simulink model "gm_HDLPayloadFull_vs"  (R2024a)
settings: Solver=FixedStepDiscrete  StartTime=0.0  StopTime=stopTime  RelTol=1e-3
values from neighbouring files (symbols this model uses):
  blockSize = logical([0 0])    [testPayloadFull.m]
  dataChars = uint8(zeros(payloadLenInWords, 1))    [testPayloadFull.m]
  fecRate = logical([1 0 0])    [testPayloadFull.m]
  fs = 1    [testPayloadFull.m]
  scramblerInit = logical([1 1 0 0])    [testPayloadFull.m]
undefined symbols (not defined in the file or in its folder): batId, clk, clk_enable, numDataCarriers, payloadWordsPerBlock0, psduSize, repNumber, reset_x
libraries: hdlmdlgenlib x65, hdlsllib x39, simulink x7, whdlutilities x4, dspsrcs4 x2, whdledac x1, vivadosimlib x1
settings Model: Creator=cotti  LastModifiedBy=cotti
settings OptimizationCC: BlockReduction=off  ConditionallyExecuteInputs=off  DefaultParameterBehavior=Inlined  InheritOutputTypeSmallerThanSingle=on
settings DebuggingCC: AlgebraicLoopMsg=error  ArtificialAlgebraicLoopMsg=error  InheritedTsInSrcMsg=none  SingleTaskRateTransMsg=error  UnconnectedInputMsg=warning  UnconnectedOutputMsg=warning  UnconnectedLineMsg=warning
settings HardwareCC: ProdBitPerPointer=32  ProdBitPerSizeT=32  ProdBitPerPtrDiffT=32  ProdLargestAtomicFloat=None  ProdIntDivRoundTo=Undefined  ProdEndianess=Unspecified  ProdWordSize=32  ProdHWDeviceType=ASIC/FPGA->ASIC/FPGA  TargetBitPerLong=64  TargetBitPerPointer=64  TargetBitPerSizeT=64  TargetBitPerPtrDiffT=64  TargetLongLongMode=on  TargetIntDivRoundTo=Zero  TargetEndianess=LittleEndian  TargetWordSize=64  TargetHWDeviceType=Custom Processor->MATLAB Host Computer  ProdEqTarget=off

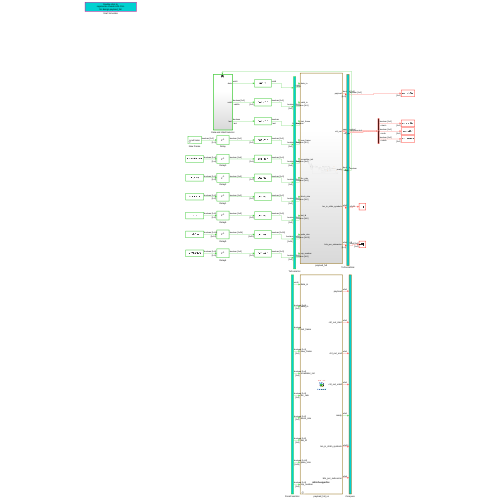
[thumbnail: Simulink's stored preview of the top-level diagram]
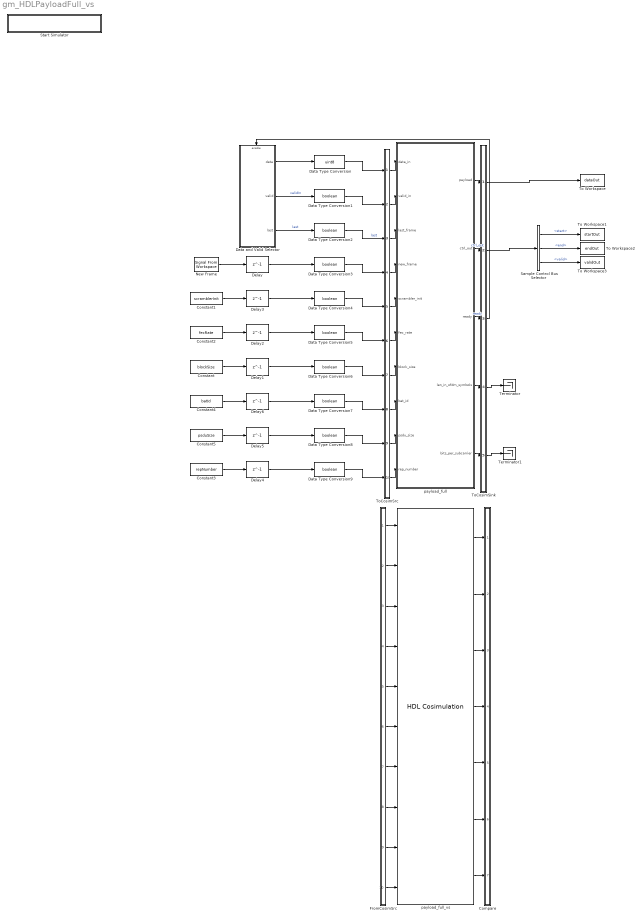
== system gm_HDLPayloadFull_vs ==
  Compare : Subsystem
      mask Display: disp('')
  Constant : Constant  Value=blockSize  VectorParams1D=off  OutDataTypeStr=boolean  SampleTime=1/fs
  Constant1 : Constant  Value=scramblerInit  VectorParams1D=off  OutDataTypeStr=boolean  SampleTime=1/fs
  Constant2 : Constant  Value=fecRate  VectorParams1D=off  OutDataTypeStr=boolean  SampleTime=1/fs
  Constant3 : Constant  Value=repNumber  VectorParams1D=off  OutDataTypeStr=boolean  SampleTime=1/fs
  Constant4 : Constant  Value=batId  VectorParams1D=off  OutDataTypeStr=boolean  SampleTime=1/fs
  Constant5 : Constant  Value=psduSize  VectorParams1D=off  OutDataTypeStr=boolean  SampleTime=1/fs
  Data Type Conversion : DataTypeConversion  OutDataTypeStr=uint8  SaturateOnIntegerOverflow=off  RndMeth=Floor
  Data Type Conversion{1..9} (9 alike) : DataTypeConversion  OutDataTypeStr=boolean  SaturateOnIntegerOverflow=off  RndMeth=Floor
  Data and Valid Selector : Subsystem  TreatAsAtomicUnit=on
  Delay{,1..6} (7 alike) : Delay  DelayLength=1  InitialCondition=0  UseCircularBuffer=on
  FromCosimSrc : Subsystem
      mask Display: disp('')
  New Frame : dspsrcs4/Signal From Workspace  X=newFrame  Ts=1/fs  nsamps=1  OutputAfterFinalValue=Setting to zero  ignoreOrWarnInputAndFrameLengths=off  OutputFrames=off
  Sample Control Bus Selector : whdlutilities/Sample Control Bus Selector  OutputSignals=start,end,valid
  Start Simulator : Subsystem
      settings: OpenFcn=|
      | cosimDirName = pwd;
      | cd 'hdl_prj/hdlsrc/HDLPayloadFull';
      | [s,r] = system('vivado -mode batch -source gm_HDLPayloadFull_vs.tcl','-echo');
      | cd (cosimDirName);
      | clear cosimDirName;
      | if s
      |    error('Failed to create Vivado HDL design DLL using script gm_HDLPayloadFull_vs.tcl.');
      | end
      mask Display: disp('Double-click to\nregenerate Vivado HDL DLL\nfor design payload_full')
  Terminator : Terminator
  Terminator1 : Terminator
  To Workspace : ToWorkspace  VariableName=dataOut  SampleTime=1/(8*fs)
      settings: Save2DSignal=2-D array (concatenate along first dimension)
  To Workspace1 : ToWorkspace  VariableName=startOut  SampleTime=1/(8*fs)
      settings: Save2DSignal=2-D array (concatenate along first dimension)
  To Workspace2 : ToWorkspace  VariableName=endOut  SampleTime=1/(8*fs)
      settings: Save2DSignal=2-D array (concatenate along first dimension)
  To Workspace3 : ToWorkspace  VariableName=validOut  SampleTime=1/(8*fs)
      settings: Save2DSignal=2-D array (concatenate along first dimension)
  ToCosimSink : Subsystem
      mask Display: disp('')
  ToCosimSrc : Subsystem
      mask Display: disp('')
  payload_full : Subsystem
  payload_full_vs : vivadosimlib/HDL Cosimulation  PortPaths=/payload_full/data_in;/payload_full/valid_in;/payload_full/last_frame;/payload_full/new_frame;/payload_full/scrambler_init;/payload_full/fec_rate;/payload_full/block_size;/payload_full/bat_id;/payload_full/psdu_size;/payload_full/rep_number;/payload_full/payload;/payload_full/ctrl_out_start;/payload_full/ctrl_out_end;/payload_full/ctrl_out_valid;/payload_full/ready;/payload_full/len_in_ofdm_symbols;/payload_full/bits_per_subcarrier  PortModes=[1 1 1 1 1 1 1 1 1 1 2 2 2 2 2 2 2 ]  PortTimes=[-1 -1 -1 -1 -1 -1 -1 -1 -1 -1 0.125 0.125 0.125 0.125 1 0.125 0.125 ]  PortSigns=[-1 -1 -1 -1 -1 -1 -1 -1 -1 -1 0 0 0 0 0 0 0 ]  PortFracLengths=[0,0,0,0,0,0,0,0,0,0,0,0,0,0,0,0,0]  PortWordLengths=[-1,-1,-1,-1,-1,-1,-1,-1,-1,-1,1,1,1,1,1,29,4]  PortHDLWordSizes=[8,1,1,1,1,1,1,1,1,1,1,1,1,1,1,29,4]  CommLocal=on  CommSharedMemory=on  CommPortNumber=4449  CommShowInfo=on  ClockPaths=clk;clk_enable;reset_x;  ClockModes=[2 4 3]  ClockTimes=[1e-08 3.7e-08 2.7e-08]  TclPostSimCommand="puts \"done\""  TimingMode=ns  TimingScaleFactor=80  idxCellArray={'UNUSED_VAR'}  CosimBypass=Full Simulation  AllowDirectFeedthrough=on  ProductName=EDA Simulator Link VS  RunAutoTimescale=off  HdlClocks=0  PreRunTime=40  PreRunTimeUnit=ns
  wires:
  Constant3/1 -> Delay4/1
  Delay1/1 -> Data Type Conversion6/1
  Sample Control Bus Selector/1 -> To Workspace1/1  "<start>"
  Constant5/1 -> Delay5/1
  New Frame/1 -> Delay/1
  Sample Control Bus Selector/3 -> To Workspace3/1  "<valid>"
  Sample Control Bus Selector/2 -> To Workspace2/1  "<end>"
  Delay5/1 -> Data Type Conversion8/1
  Constant4/1 -> Delay6/1
  Delay2/1 -> Data Type Conversion5/1
  Data and Valid Selector/3(last) -> Data Type Conversion2/1  "last"
  Constant2/1 -> Delay2/1
  Delay3/1 -> Data Type Conversion4/1
  Constant1/1 -> Delay3/1
  Delay/1 -> Data Type Conversion3/1
  Data and Valid Selector/1(data) -> Data Type Conversion/1
  Data and Valid Selector/2(valid) -> Data Type Conversion1/1  "validIn"
  Delay4/1 -> Data Type Conversion9/1
  Constant/1 -> Delay1/1
  Delay6/1 -> Data Type Conversion7/1
  ToCosimSrc/1(out1) -> payload_full/1(data_in)
  ToCosimSrc/2(out2) -> payload_full/2(valid_in)
  ToCosimSrc/3(out3) -> payload_full/3(last_frame)
  ToCosimSrc/4(out4) -> payload_full/4(new_frame)
  ToCosimSrc/5(out5) -> payload_full/5(scrambler_init)
  ToCosimSrc/6(out6) -> payload_full/6(fec_rate)
  ToCosimSrc/7(out7) -> payload_full/7(block_size)
  ToCosimSrc/8(out8) -> payload_full/8(bat_id)
  ToCosimSrc/9(out9) -> payload_full/9(psdu_size)
  ToCosimSrc/10(out10) -> payload_full/10(rep_number)
  payload_full/1(payload) -> ToCosimSink/1(in1)
  payload_full/2(ctrl_out) -> ToCosimSink/2(in2)  "ctrl_out"
  payload_full/3(ready) -> ToCosimSink/3(in3)  "ready"
  payload_full/4(len_in_ofdm_symbols) -> ToCosimSink/4(in4)
  payload_full/5(bits_per_subcarrier) -> ToCosimSink/5(in5)
  Data Type Conversion/1 -> ToCosimSrc/1(in1)
  Data Type Conversion1/1 -> ToCosimSrc/2(in2)
  Data Type Conversion2/1 -> ToCosimSrc/3(in3)  "last"
  Data Type Conversion3/1 -> ToCosimSrc/4(in4)
  Data Type Conversion4/1 -> ToCosimSrc/5(in5)
  Data Type Conversion5/1 -> ToCosimSrc/6(in6)
  Data Type Conversion6/1 -> ToCosimSrc/7(in7)
  Data Type Conversion7/1 -> ToCosimSrc/8(in8)
  Data Type Conversion8/1 -> ToCosimSrc/9(in9)
  Data Type Conversion9/1 -> ToCosimSrc/10(in10)
  ToCosimSink/1(out1) -> To Workspace/1
  ToCosimSink/2(out2) -> Sample Control Bus Selector/1
  ToCosimSink/3(out3) -> Data and Valid Selector/Enable
  ToCosimSink/4(out4) -> Terminator/1
  ToCosimSink/5(out5) -> Terminator1/1
  FromCosimSrc/1(out1) -> payload_full_vs/1
  FromCosimSrc/2(out2) -> payload_full_vs/2
  FromCosimSrc/3(out3) -> payload_full_vs/3
  FromCosimSrc/4(out4) -> payload_full_vs/4
  FromCosimSrc/5(out5) -> payload_full_vs/5
  FromCosimSrc/6(out6) -> payload_full_vs/6
  FromCosimSrc/7(out7) -> payload_full_vs/7
  FromCosimSrc/8(out8) -> payload_full_vs/8
  FromCosimSrc/9(out9) -> payload_full_vs/9
  FromCosimSrc/10(out10) -> payload_full_vs/10
  payload_full_vs/1 -> Compare/1(in1)
  payload_full_vs/2 -> Compare/2(in2)
  payload_full_vs/3 -> Compare/3(in3)
  payload_full_vs/4 -> Compare/4(in4)
  payload_full_vs/5 -> Compare/5(in5)
  payload_full_vs/6 -> Compare/6(in6)
  payload_full_vs/7 -> Compare/7(in7)

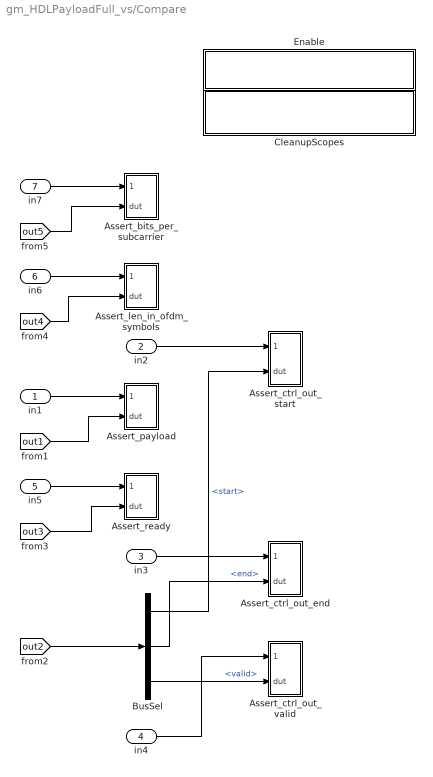
== system gm_HDLPayloadFull_vs/Compare ==
  in1 : Inport
  in2 : Inport  Port=2
  in3 : Inport  Port=3
  in4 : Inport  Port=4
  in5 : Inport  Port=5
  in6 : Inport  Port=6
  in7 : Inport  Port=7
  Assert_bits_per_subcarrier : Subsystem
      settings: LibrarySourceBlock=hdlmdlgenlib/AssertEq
  Assert_ctrl_out_end : Subsystem
      settings: LibrarySourceBlock=hdlmdlgenlib/AssertEq
  Assert_ctrl_out_start : Subsystem
      settings: LibrarySourceBlock=hdlmdlgenlib/AssertEq
  Assert_ctrl_out_valid : Subsystem
      settings: LibrarySourceBlock=hdlmdlgenlib/AssertEq
  Assert_len_in_ofdm_symbols : Subsystem
      settings: LibrarySourceBlock=hdlmdlgenlib/AssertEq
  Assert_payload : Subsystem
      settings: LibrarySourceBlock=hdlmdlgenlib/AssertEq
  Assert_ready : Subsystem
      settings: LibrarySourceBlock=hdlmdlgenlib/AssertEq
  BusSel : BusSelector  OutputSignals=start,end,valid
  CleanupScopes : Subsystem
      settings: OpenFcn=|
      | blkName = gcb; %self block
      | idx = regexp(blkName, '/CleanupScopes$', 'once');
      | blkParent = blkName(1:idx-1);
      | blks=find_system(blkParent, 'LookUnderMasks', 'all','blocktype', 'Scope');
      | for itr = 1:length(blks)
      | 	 hScopeCfg = get_param(blks{itr},'ScopeConfiguration');
      | 	 hScopeCfg.Visible = ~ hScopeCfg.Visible;
      | end
      | drawnow;
      mask Display: fprintf(message('hdlcoder:cosim:vnl_dblclick').getString());
  Enable : Subsystem
      settings: OpenFcn=|
      | blkName = gcb;
      | idx = regexp(blkName, '/Enable$', 'once');
      | blkParent = blkName(1:idx-1);
      | blks=find_system(blkParent, 'LookUnderMasks', 'all','blocktype', 'Assertion');
      | e = get_param(blks{1}, 'Enabled');
      | if strcmp(e, 'on'), f= 'off';, else, f = 'on';, end
      | for ii=1:length(blks), set_param(blks{ii}, 'Enabled', f);, end
      | set_param(gcb, 'MaskDisplay',['fprintf(message(''hdlcoder:cosim:vnl_dblclick_assertions'',','''',upper(e),'''',').getString())']);
      mask Display: fprintf(message('hdlcoder:cosim:vnl_dblclick_assertions','OFF').getString());
  wires:
  in4/1 -> Assert_ctrl_out_valid/1(cosim)
  in6/1 -> Assert_len_in_ofdm_symbols/1(cosim)
  in7/1 -> Assert_bits_per_subcarrier/1(cosim)
  [out5] -> Assert_bits_per_subcarrier/2(dut)
  [out4] -> Assert_len_in_ofdm_symbols/2(dut)
  in1/1 -> Assert_payload/1(cosim)
  in5/1 -> Assert_ready/1(cosim)
  [out1] -> Assert_payload/2(dut)
  [out3] -> Assert_ready/2(dut)
  [out2] -> BusSel/1
  BusSel/1 -> Assert_ctrl_out_start/2(dut)  "<start>"
  BusSel/3 -> Assert_ctrl_out_valid/2(dut)  "<valid>"
  BusSel/2 -> Assert_ctrl_out_end/2(dut)  "<end>"
  in2/1 -> Assert_ctrl_out_start/1(cosim)
  in3/1 -> Assert_ctrl_out_end/1(cosim)

== system gm_HDLPayloadFull_vs/Data and Valid Selector ==
  note: This subsystem is active only when the input ready signal is active. The subsystem selects the Input Valid value and outputs the valid signal.
      | The subsystem also selects the payload data from an LUT based on the Input Valid signal and outputs it as data signal.
  Enable : EnablePort
  Direct Lookup Table (n-D) : LookupNDDirect  NumberOfTableDimensions=1  Table=dataChars  DiagnosticForOutOfRangeInput=Error  TableDataTypeStr=uint8
  HDL Counter : hdlsllib/Sources/HDL Counter  CountType=Count limited  CountInit=0  CountStep=1  CountMax=length(dataChars) -1  CountFromType=Initial value  CountFrom=0  CountResetPort=off  CountLoadPort=off  CountEnbPort=on  CountDirPort=off  CountHitOutputPort=on  CountDataType=Unsigned  CountWordLen=nextpow2(length(dataChars))  CountFracLen=0  CountSampTime=1
  Input Valid : dspsrcs4/Signal From Workspace  X=validIn  Ts=1/fs  nsamps=1  OutputAfterFinalValue=Setting to zero  ignoreOrWarnInputAndFrameLengths=off  OutputFrames=off
  data : Outport  InitialOutput=0  VectorParamsAs1DForOutWhenUnconnected=off
  valid : Outport  Port=2  InitialOutput=0  VectorParamsAs1DForOutWhenUnconnected=off
  last : Outport  Port=3  VectorParamsAs1DForOutWhenUnconnected=off
  wires:
  HDL Counter/1 -> Direct Lookup Table (n-D)/1
  Direct Lookup Table (n-D)/1 -> data/1
  HDL Counter/2 -> last/1
  Input Valid/1 -> valid/1, HDL Counter/1

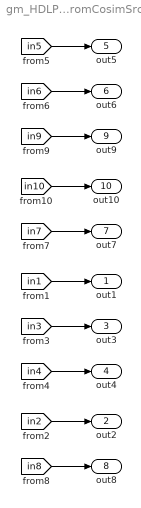
== system gm_HDLPayloadFull_vs/FromCosimSrc ==
  out1 : Outport
  out2 : Outport  Port=2
  out3 : Outport  Port=3
  out4 : Outport  Port=4
  out5 : Outport  Port=5
  out6 : Outport  Port=6
  out7 : Outport  Port=7
  out8 : Outport  Port=8
  out9 : Outport  Port=9
  out10 : Outport  Port=10
  wires:
  [in4] -> out4/1
  [in3] -> out3/1
  [in7] -> out7/1
  [in10] -> out10/1
  [in8] -> out8/1
  [in9] -> out9/1
  [in2] -> out2/1
  [in1] -> out1/1
  [in6] -> out6/1
  [in5] -> out5/1

== system gm_HDLPayloadFull_vs/Start Simulator ==

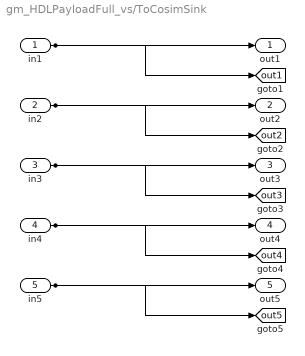
== system gm_HDLPayloadFull_vs/ToCosimSink ==
  in1 : Inport
  in2 : Inport  Port=2
  in3 : Inport  Port=3
  in4 : Inport  Port=4
  in5 : Inport  Port=5
  out1 : Outport
  out2 : Outport  Port=2
  out3 : Outport  Port=3
  out4 : Outport  Port=4
  out5 : Outport  Port=5
  tag scope: out1=global, out2=global, out3=global, out4=global, out5=global
  wires:
  in1/1 -> out1/1, [out1]
  in2/1 -> out2/1, [out2]
  in3/1 -> out3/1, [out3]
  in4/1 -> out4/1, [out4]
  in5/1 -> out5/1, [out5]

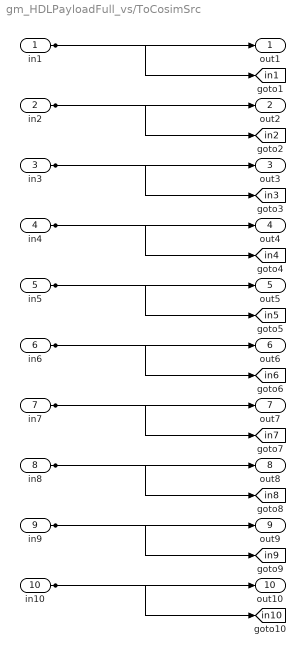
== system gm_HDLPayloadFull_vs/ToCosimSrc ==
  in1 : Inport
  in2 : Inport  Port=2
  in3 : Inport  Port=3
  in4 : Inport  Port=4
  in5 : Inport  Port=5
  in6 : Inport  Port=6
  in7 : Inport  Port=7
  in8 : Inport  Port=8
  in9 : Inport  Port=9
  in10 : Inport  Port=10
  out1 : Outport
  out2 : Outport  Port=2
  out3 : Outport  Port=3
  out4 : Outport  Port=4
  out5 : Outport  Port=5
  out6 : Outport  Port=6
  out7 : Outport  Port=7
  out8 : Outport  Port=8
  out9 : Outport  Port=9
  out10 : Outport  Port=10
  tag scope: in10=global, in1=global, in2=global, in3=global, in4=global, in5=global, in6=global, in7=global, in8=global, in9=global
  wires:
  in1/1 -> out1/1, [in1]
  in2/1 -> out2/1, [in2]
  in3/1 -> out3/1, [in3]
  in4/1 -> out4/1, [in4]
  in5/1 -> out5/1, [in5]
  in6/1 -> out6/1, [in6]
  in7/1 -> out7/1, [in7]
  in8/1 -> out8/1, [in8]
  in9/1 -> out9/1, [in9]
  in10/1 -> out10/1, [in10]

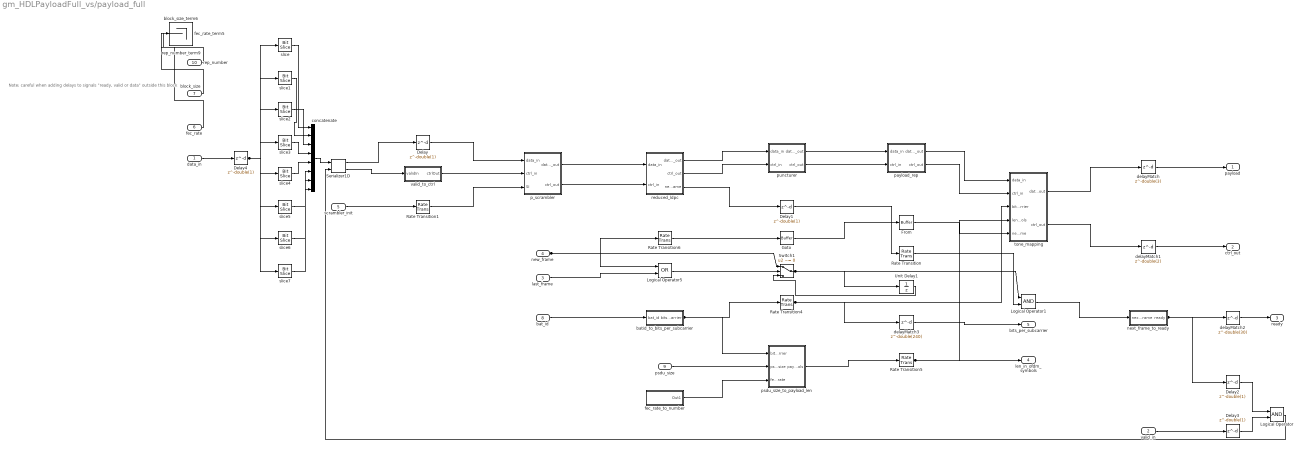
== system gm_HDLPayloadFull_vs/payload_full ==
  note: Note: careful when adding delays to signals "ready, valid or data" outside this block
  data_in : Inport  OutDataTypeStr=uint8  SampleTime=1
  valid_in : Inport  Port=2  OutDataTypeStr=boolean  SampleTime=1
  last_frame : Inport  Port=3  OutDataTypeStr=boolean  SampleTime=1
  new_frame : Inport  Port=4  OutDataTypeStr=boolean  SampleTime=1
  scrambler_init : Inport  Port=5  OutDataTypeStr=boolean  PortDimensions=[1 4]  SampleTime=1
  fec_rate : Inport  Port=6  OutDataTypeStr=boolean  PortDimensions=[1 3]  SampleTime=1
  block_size : Inport  Port=7  OutDataTypeStr=boolean  PortDimensions=[1 2]  SampleTime=1
  bat_id : Inport  Port=8  OutDataTypeStr=boolean  PortDimensions=[1 5]  SampleTime=1
  psdu_size : Inport  Port=9  OutDataTypeStr=boolean  PortDimensions=[1 24]  SampleTime=1
  rep_number : Inport  Port=10  OutDataTypeStr=boolean  PortDimensions=[1 3]  SampleTime=1
  Delay : Delay  DelayLength=double(1)  InitialCondition=0  SampleTime=0.125
  Delay1 : Delay  DelayLength=double(1)  InitialCondition=0  SampleTime=0.125
  Delay2 : Delay  DelayLength=double(1)  InitialCondition=0  SampleTime=1
  Delay3 : Delay  DelayLength=double(1)  InitialCondition=0  SampleTime=1
  Delay4 : Delay  DelayLength=double(1)  InitialCondition=0  SampleTime=1
  From : hdlmdlgenlib/Buffer
  Goto : hdlmdlgenlib/Buffer
  Logical Operator : Logic  AllPortsSameDT=off  OutDataTypeStr=boolean  SampleTime=1
  Logical Operator1 : Logic  AllPortsSameDT=off  OutDataTypeStr=boolean  SampleTime=1
  Logical Operator5 : Logic  Operator=OR  AllPortsSameDT=off  OutDataTypeStr=boolean  SampleTime=1
  Rate Transition : RateTransition  InitialCondition=double(0)  OutPortSampleTimeOpt=Multiple of input port sample time  OutPortSampleTimeMultiple=8
  Rate Transition1 : RateTransition  OutPortSampleTimeOpt=Multiple of input port sample time  OutPortSampleTimeMultiple=1/8
  Rate Transition4 : RateTransition  InitialCondition="fi(0,0,4,0,\"hex\",\"0\")"  OutPortSampleTimeOpt=Multiple of input port sample time  OutPortSampleTimeMultiple=1/8
  Rate Transition5 : RateTransition  InitialCondition="fi(0,0,29,0,\"hex\",\"00000000\")"  OutPortSampleTimeOpt=Multiple of input port sample time  OutPortSampleTimeMultiple=1/8
  Rate Transition6 : RateTransition  OutPortSampleTimeOpt=Multiple of input port sample time  OutPortSampleTimeMultiple=1/8
  Serializer1D : hdlsllib/HDL Operations/Serializer1D  Ratio=8  IdleCycles=0  validIn=on  startOut=off  validOut=on  inputDataDimensions=8  inputSampleTime=1  inputSignalType=real
  Switch1 : Switch  Criteria=u2 ~= 0  Threshold=double(0)  OutDataTypeStr=boolean  SampleTime=1  SaturateOnIntegerOverflow=off  InputSameDT=off
  Unit Delay1 : UnitDelay  SampleTime=1
  batid_to_bits_per_subcarrier : Subsystem
  block_size_term6 : Terminator
  concatenate : Concatenate  NumInputs=8  Mode=Multidimensional array  ConcatenateDimension=2
  delayMatch : Delay  DelayLength=double(3)  InitialCondition=0  SampleTime=0.125
  delayMatch1 : Delay  DelayLength=double(2)  InitialCondition=0  SampleTime=0.125
  delayMatch2 : Delay  DelayLength=double(30)  InitialCondition=0  SampleTime=1
  delayMatch3 : Delay  DelayLength=double(240)  InitialCondition=0  SampleTime=0.125
  fec_rate_term5 : Terminator
  fec_rate_to_number : Subsystem
  next_frame_to_ready : Subsystem
  p_scrambler : Subsystem
  payload_rep : Subsystem
  psdu_size_to_payload_len : Subsystem
  puncturer : Subsystem
  reduced_ldpc : Subsystem
  rep_number_term9 : Terminator
  slice : hdlsllib/Logic and Bit Operations/Bit Slice  lidx=double(0)  ridx=double(0)
  slice1 : hdlsllib/Logic and Bit Operations/Bit Slice  lidx=double(1)  ridx=double(1)
  slice2 : hdlsllib/Logic and Bit Operations/Bit Slice  lidx=double(2)  ridx=double(2)
  slice3 : hdlsllib/Logic and Bit Operations/Bit Slice  lidx=double(3)  ridx=double(3)
  slice4 : hdlsllib/Logic and Bit Operations/Bit Slice  lidx=double(4)  ridx=double(4)
  slice5 : hdlsllib/Logic and Bit Operations/Bit Slice  lidx=double(5)  ridx=double(5)
  slice6 : hdlsllib/Logic and Bit Operations/Bit Slice  lidx=double(6)  ridx=double(6)
  slice7 : hdlsllib/Logic and Bit Operations/Bit Slice  lidx=double(7)  ridx=double(7)
  tone_mapping : Subsystem
  valid_to_ctrl : Subsystem
  payload : Outport  SampleTime=0.125
  ctrl_out : Outport  Port=2  SampleTime=0.125
  ready : Outport  Port=3  SampleTime=1
  len_in_ofdm_symbols : Outport  Port=4  SampleTime=0.125
  bits_per_subcarrier : Outport  Port=5  SampleTime=0.125
  wires:
  Rate Transition/1 -> Logical Operator1/2
  Logical Operator1/1 -> next_frame_to_ready/1(next_frame)
  reduced_ldpc/3(next_frame) -> Delay1/1
  Logical Operator/1 -> Serializer1D/2
  Serializer1D/2 -> valid_to_ctrl/1(validIn)
  Serializer1D/1 -> Delay/1
  Delay2/1 -> Logical Operator/1
  Rate Transition1/1 -> p_scrambler/3(SI)
  p_scrambler/2(ctrl_out) -> reduced_ldpc/2(ctrl_in)
  Delay3/1 -> Logical Operator/2
  valid_to_ctrl/1(ctrlOut) -> p_scrambler/2(ctrl_in)
  Delay1/1 -> Rate Transition/1
  p_scrambler/1(data_out) -> reduced_ldpc/1(data_in)
  Delay/1 -> p_scrambler/1(data_in)
  Logical Operator5/1 -> Switch1/2
  Unit Delay1/1 -> Switch1/3
  Rate Transition4/1 -> tone_mapping/3(bits_per_subcarrier), delayMatch3/1
  next_frame_to_ready/1(ready) -> Delay2/1, delayMatch2/1
  tone_mapping/2(ctrl_out) -> delayMatch1/1
  tone_mapping/1(data_out) -> delayMatch/1
  slice7/1 -> concatenate/8
  slice6/1 -> concatenate/7
  slice5/1 -> concatenate/6
  slice4/1 -> concatenate/5
  slice3/1 -> concatenate/4
  slice2/1 -> concatenate/3
  slice1/1 -> concatenate/2
  slice/1 -> concatenate/1
  Goto/1 -> From/1
  delayMatch1/1 -> ctrl_out/1
  delayMatch/1 -> payload/1
  reduced_ldpc/2(ctrl_out) -> puncturer/2(ctrl_in)
  reduced_ldpc/1(data_out) -> puncturer/1(data_in)
  puncturer/2(ctrl_out) -> payload_rep/2(ctrl_in)
  puncturer/1(data_out) -> payload_rep/1(data_in)
  psdu_size_to_payload_len/1(payload_len_in_ofdm_symbols) -> Rate Transition5/1
  payload_rep/2(ctrl_out) -> tone_mapping/2(ctrl_in)
  payload_rep/1(data_out) -> tone_mapping/1(data_in)
  delayMatch2/1 -> ready/1
  fec_rate_to_number/1(Out1) -> psdu_size_to_payload_len/3(fec_rate)
  batid_to_bits_per_subcarrier/1(bits_per_subcarrier) -> psdu_size_to_payload_len/1(bits_per_subcarrier), Rate Transition4/1
  concatenate/1 -> Serializer1D/1
  Switch1/1 -> Logical Operator1/1, Unit Delay1/1
  Rate Transition6/1 -> Goto/1
  Rate Transition5/1 -> tone_mapping/4(len_in_ofdm_symbols), len_in_ofdm_symbols/1
  delayMatch3/1 -> bits_per_subcarrier/1
  From/1 -> tone_mapping/5(new_frame)
  Delay4/1 -> slice/1, slice1/1, slice2/1, slice3/1, slice4/1, slice5/1, slice6/1, slice7/1
  rep_number/1 -> rep_number_term9/1
  psdu_size/1 -> psdu_size_to_payload_len/2(psdu_size)
  bat_id/1 -> batid_to_bits_per_subcarrier/1(bat_id)
  block_size/1 -> block_size_term6/1
  fec_rate/1 -> fec_rate_term5/1
  scrambler_init/1 -> Rate Transition1/1
  new_frame/1 -> Switch1/1, Rate Transition6/1, Logical Operator5/1
  last_frame/1 -> Logical Operator5/2
  valid_in/1 -> Delay3/1
  data_in/1 -> Delay4/1

== system gm_HDLPayloadFull_vs/Compare/Assert_bits_per_subcarrier ==
  cosim : Inport
  dut : Inport  Port=2
  AssertEq : Assertion
  Compare To Zero : simulink/Logic and Bit Operations/Compare To Zero  relop===  OutDataTypeStr=boolean
  Relational Operator : RelationalOperator  Operator===  OutDataTypeStr=boolean  InputSameDT=off
  compare: bits_per_subcarrier : Scope  NumInputPorts=3
  wires:
  Compare To Zero/1 -> compare: bits_per_subcarrier/3  "err"
  Relational Operator/1 -> Compare To Zero/1, AssertEq/1
  cosim/1 -> compare: bits_per_subcarrier/1, Relational Operator/1  "cosim"
  dut/1 -> compare: bits_per_subcarrier/2, Relational Operator/2  "dut ref"

== system gm_HDLPayloadFull_vs/Compare/Assert_ctrl_out_end ==
  cosim : Inport
  dut : Inport  Port=2
  AssertEq : Assertion
  Compare To Zero : simulink/Logic and Bit Operations/Compare To Zero  relop===  OutDataTypeStr=boolean
  Relational Operator : RelationalOperator  Operator===  OutDataTypeStr=boolean  InputSameDT=off
  compare: ctrl_out : Scope  NumInputPorts=3
  wires:
  Compare To Zero/1 -> compare: ctrl_out/3  "err"
  Relational Operator/1 -> Compare To Zero/1, AssertEq/1
  cosim/1 -> compare: ctrl_out/1, Relational Operator/1  "cosim"
  dut/1 -> compare: ctrl_out/2, Relational Operator/2  "dut ref"

== system gm_HDLPayloadFull_vs/Compare/Assert_ctrl_out_start ==
  cosim : Inport
  dut : Inport  Port=2
  AssertEq : Assertion
  Compare To Zero : simulink/Logic and Bit Operations/Compare To Zero  relop===  OutDataTypeStr=boolean
  Relational Operator : RelationalOperator  Operator===  OutDataTypeStr=boolean  InputSameDT=off
  compare: ctrl_out : Scope  NumInputPorts=3
  wires:
  Compare To Zero/1 -> compare: ctrl_out/3  "err"
  Relational Operator/1 -> Compare To Zero/1, AssertEq/1
  cosim/1 -> compare: ctrl_out/1, Relational Operator/1  "cosim"
  dut/1 -> compare: ctrl_out/2, Relational Operator/2  "dut ref"

== system gm_HDLPayloadFull_vs/Compare/Assert_ctrl_out_valid ==
  cosim : Inport
  dut : Inport  Port=2
  AssertEq : Assertion
  Compare To Zero : simulink/Logic and Bit Operations/Compare To Zero  relop===  OutDataTypeStr=boolean
  Relational Operator : RelationalOperator  Operator===  OutDataTypeStr=boolean  InputSameDT=off
  compare: ctrl_out : Scope  NumInputPorts=3
  wires:
  Compare To Zero/1 -> compare: ctrl_out/3  "err"
  Relational Operator/1 -> Compare To Zero/1, AssertEq/1
  cosim/1 -> compare: ctrl_out/1, Relational Operator/1  "cosim"
  dut/1 -> compare: ctrl_out/2, Relational Operator/2  "dut ref"

== system gm_HDLPayloadFull_vs/Compare/Assert_len_in_ofdm_symbols ==
  cosim : Inport
  dut : Inport  Port=2
  AssertEq : Assertion
  Compare To Zero : simulink/Logic and Bit Operations/Compare To Zero  relop===  OutDataTypeStr=boolean
  Relational Operator : RelationalOperator  Operator===  OutDataTypeStr=boolean  InputSameDT=off
  compare: len_in_ofdm_symbols : Scope  NumInputPorts=3
  wires:
  Compare To Zero/1 -> compare: len_in_ofdm_symbols/3  "err"
  Relational Operator/1 -> Compare To Zero/1, AssertEq/1
  cosim/1 -> compare: len_in_ofdm_symbols/1, Relational Operator/1  "cosim"
  dut/1 -> compare: len_in_ofdm_symbols/2, Relational Operator/2  "dut ref"

== system gm_HDLPayloadFull_vs/Compare/Assert_payload ==
  cosim : Inport
  dut : Inport  Port=2
  AssertEq : Assertion
  Compare To Zero : simulink/Logic and Bit Operations/Compare To Zero  relop===  OutDataTypeStr=boolean
  Relational Operator : RelationalOperator  Operator===  OutDataTypeStr=boolean  InputSameDT=off
  compare: payload : Scope  NumInputPorts=3
  wires:
  Compare To Zero/1 -> compare: payload/3  "err"
  Relational Operator/1 -> Compare To Zero/1, AssertEq/1
  cosim/1 -> compare: payload/1, Relational Operator/1  "cosim"
  dut/1 -> compare: payload/2, Relational Operator/2  "dut ref"

== system gm_HDLPayloadFull_vs/Compare/Assert_ready ==
  cosim : Inport
  dut : Inport  Port=2
  AssertEq : Assertion
  Compare To Zero : simulink/Logic and Bit Operations/Compare To Zero  relop===  OutDataTypeStr=boolean
  Relational Operator : RelationalOperator  Operator===  OutDataTypeStr=boolean  InputSameDT=off
  compare: ready : Scope  NumInputPorts=3
  wires:
  Compare To Zero/1 -> compare: ready/3  "err"
  Relational Operator/1 -> Compare To Zero/1, AssertEq/1
  cosim/1 -> compare: ready/1, Relational Operator/1  "cosim"
  dut/1 -> compare: ready/2, Relational Operator/2  "dut ref"

== system gm_HDLPayloadFull_vs/Compare/CleanupScopes ==

== system gm_HDLPayloadFull_vs/Compare/Enable ==

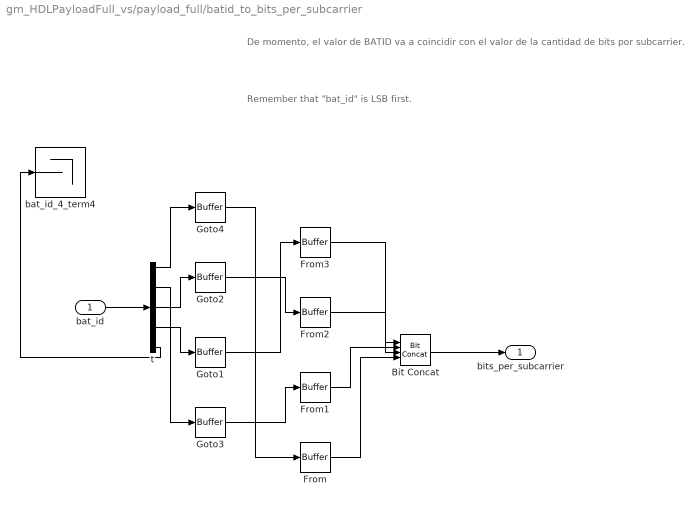
== system gm_HDLPayloadFull_vs/payload_full/batid_to_bits_per_subcarrier ==
  note: Remember that "bat_id" is LSB first.
  note: De momento, el valor de BATID va a coincidir con el valor de la cantidad de bits por subcarrier.
  bat_id : Inport  OutDataTypeStr=boolean  PortDimensions=[1 5]  SampleTime=1
  Bit Concat : hdlsllib/Logic and Bit Operations/Bit Concat  numInputs=4
  From{,1..3} (4 alike) : hdlmdlgenlib/Buffer
  Goto{1..4} (4 alike) : hdlmdlgenlib/Buffer
  bat_id_4_term4 : Terminator
  t : Demux  Outputs=5
  bits_per_subcarrier : Outport  SampleTime=1
  wires:
  t/5 -> bat_id_4_term4/1
  t/4 -> Goto1/1
  t/3 -> Goto2/1
  t/2 -> Goto3/1
  t/1 -> Goto4/1
  Goto1/1 -> From3/1
  Goto2/1 -> From2/1
  Goto3/1 -> From1/1
  Goto4/1 -> From/1
  From3/1 -> Bit Concat/1
  From2/1 -> Bit Concat/2
  From1/1 -> Bit Concat/3
  From/1 -> Bit Concat/4
  Bit Concat/1 -> bits_per_subcarrier/1
  bat_id/1 -> t/1

== system gm_HDLPayloadFull_vs/payload_full/fec_rate_to_number ==
  Constant : Constant  Value=2  OutDataTypeStr=fixdt(0,4,0)  SampleTime=-1
  Out1 : Outport  SampleTime=1
  wires:
  Constant/1 -> Out1/1

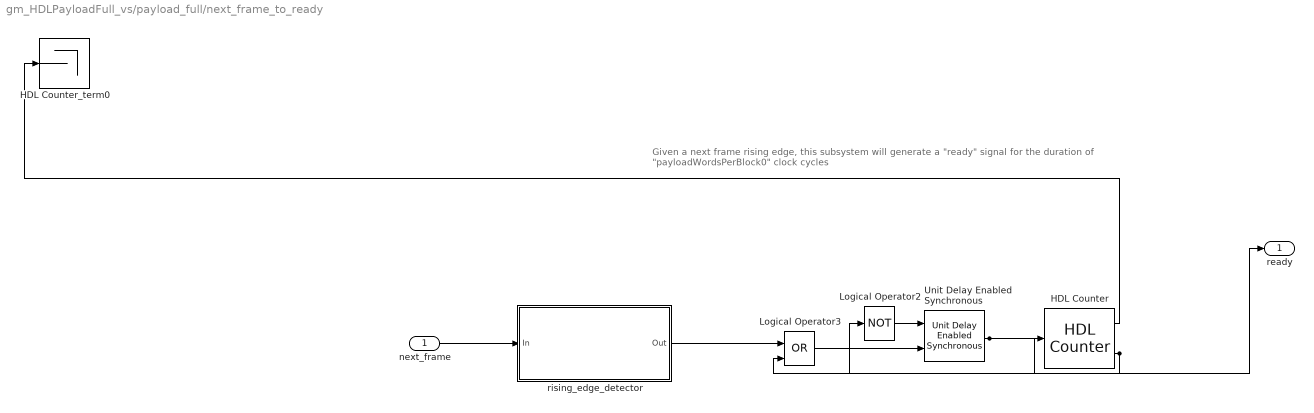
== system gm_HDLPayloadFull_vs/payload_full/next_frame_to_ready ==
  note: Given a next frame rising edge, this subsystem will generate a "ready" signal for the duration of "payloadWordsPerBlock0" clock cycles
  next_frame : Inport  OutDataTypeStr=boolean  SampleTime=1
  HDL Counter : hdlsllib/Sources/HDL Counter  CountType=Count limited  CountInit=0  CountStep=1  CountMax=payloadWordsPerBlock0-1  CountFromType=Initial value  CountFrom=0  CountResetPort=off  CountLoadPort=off  CountEnbPort=on  CountDirPort=off  CountHitOutputPort=on  CountDataType=Unsigned  CountWordLen=nextpow2(payloadWordsPerBlock0)  CountFracLen=0  CountSampTime=1
  HDL Counter_term0 : Terminator
  Logical Operator2 : Logic  Operator=NOT  IconShape=distinctive  AllPortsSameDT=off  OutDataTypeStr=boolean
  Logical Operator3 : Logic  Operator=OR  IconShape=distinctive  AllPortsSameDT=off  OutDataTypeStr=boolean
  Unit Delay Enabled Synchronous : hdlsllib/Discrete/Unit Delay Enabled Synchronous  InitialCondition=0.0  SampleTime=-1
  rising_edge_detector : Subsystem
  ready : Outport  SampleTime=1
  wires:
  Logical Operator2/1 -> Unit Delay Enabled Synchronous/1
  HDL Counter/2 -> Logical Operator2/1, Logical Operator3/2
  Logical Operator3/1 -> Unit Delay Enabled Synchronous/2
  rising_edge_detector/1(Out) -> Logical Operator3/1
  Unit Delay Enabled Synchronous/1 -> HDL Counter/1, ready/1
  HDL Counter/1 -> HDL Counter_term0/1
  next_frame/1 -> rising_edge_detector/1(In)

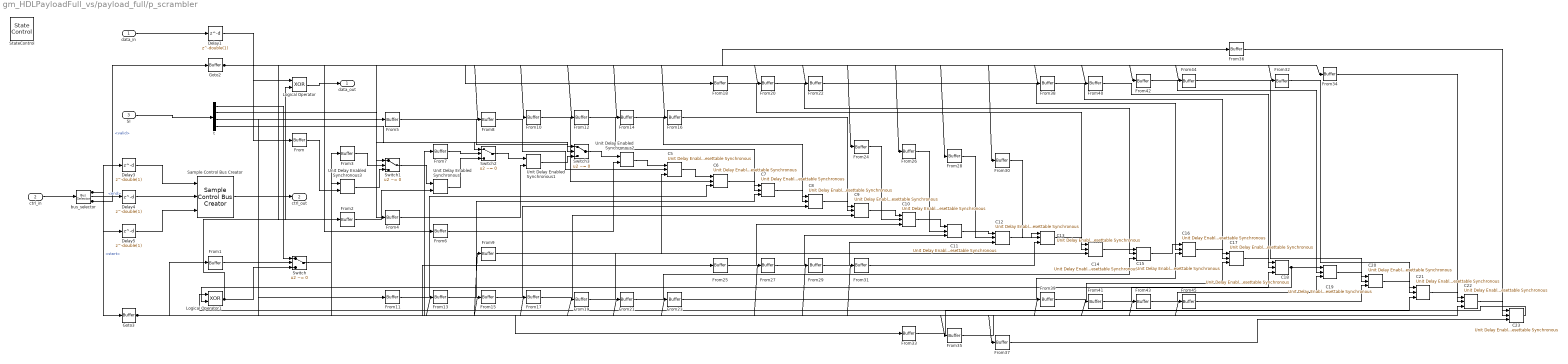
== system gm_HDLPayloadFull_vs/payload_full/p_scrambler ==
  data_in : Inport  OutDataTypeStr=fixdt(0, 1, 0)  SampleTime=0.125
  ctrl_in : Inport  Port=2  SampleTime=0.125
  SI : Inport  Port=3  OutDataTypeStr=boolean  PortDimensions=[1 4]  SampleTime=0.125
  C{5..23} (19 alike) : hdlsllib/Discrete/Unit Delay Enabled Resettable Synchronous  InitialCondition=double(1)  SampleTime=-1
  Delay{1,3..5} (4 alike) : Delay  DelayLength=double(1)  InitialCondition=0  SampleTime=0.125
  From{,1..45} (46 alike) : hdlmdlgenlib/Buffer
  Goto2 : hdlmdlgenlib/Buffer
  Goto3 : hdlmdlgenlib/Buffer
  Logical Operator : Logic  Operator=XOR  AllPortsSameDT=off  OutDataTypeStr=boolean  SampleTime=0.125
  Logical Operator1 : Logic  Operator=XOR  AllPortsSameDT=off  OutDataTypeStr=boolean  SampleTime=0.125
  Sample Control Bus Creator : whdlutilities/Sample Control Bus Creator
  StateControl : StateControl  StateControl=Synchronous
  Switch{,1..3} (4 alike) : Switch  Criteria=u2 ~= 0  Threshold=double(0)  OutDataTypeStr=boolean  SampleTime=0.125  SaturateOnIntegerOverflow=off  InputSameDT=off
  Unit Delay Enabled Synchronous{,1..3} (4 alike) : hdlsllib/Discrete/Unit Delay Enabled Synchronous  InitialCondition=double(1)  SampleTime=-1
  bus_selector : BusSelector  OutputSignals=start,end,valid
  t : Demux
  data_out : Outport  SampleTime=0.125
  ctrl_out : Outport  Port=2  SampleTime=0.125
  wires:
  C23/1 -> Logical Operator1/1
  C22/1 -> C23/1
  C21/1 -> C22/1
  C20/1 -> C21/1
  C19/1 -> C20/1
  C18/1 -> C19/1, Logical Operator1/2
  C17/1 -> C18/1
  C16/1 -> C17/1
  C15/1 -> C16/1
  C14/1 -> C15/1
  C13/1 -> C14/1
  C12/1 -> C13/1
  C11/1 -> C12/1
  C10/1 -> C11/1
  C9/1 -> C10/1
  C8/1 -> C9/1
  C7/1 -> C8/1
  C6/1 -> C7/1
  C5/1 -> C6/1
  Unit Delay Enabled Synchronous2/1 -> C5/1
  Switch3/1 -> Unit Delay Enabled Synchronous2/1
  Unit Delay Enabled Synchronous1/1 -> Switch3/3
  Switch2/1 -> Unit Delay Enabled Synchronous1/1
  Unit Delay Enabled Synchronous/1 -> Switch2/3
  Switch1/1 -> Unit Delay Enabled Synchronous/1
  Unit Delay Enabled Synchronous3/1 -> Switch1/3
  Switch/1 -> Unit Delay Enabled Synchronous3/1
  t/4 -> Switch3/1
  t/3 -> Switch2/1
  t/2 -> Switch1/1
  t/1 -> Switch/1
  Goto3/1 -> From1/1, From11/1, From13/1, From15/1, From17/1, From19/1, From21/1, From23/1, From25/1, From27/1, From29/1, From3/1, From31/1, From33/1, From35/1, From37/1, From39/1, From41/1, From43/1, From45/1, From5/1, From7/1, From9/1
  Goto2/1 -> From/1, From10/1, From12/1, From14/1, From16/1, From18/1, From2/1, From20/1, From22/1, From24/1, From26/1, From28/1, From30/1, From32/1, From34/1, From36/1, From38/1, From4/1, From40/1, From42/1, From44/1, From6/1, From8/1
  Sample Control Bus Creator/1 -> ctrl_out/1
  Logical Operator1/1 -> Switch/3, Logical Operator/2
  Logical Operator/1 -> data_out/1
  From9/1 -> C5/3
  From8/1 -> C5/2
  From7/1 -> Switch2/2
  From6/1 -> Unit Delay Enabled Synchronous2/2
  From5/1 -> Switch3/2
  From45/1 -> C20/3
  From44/1 -> C20/2
  From43/1 -> C19/3
  From42/1 -> C19/2
  From41/1 -> C18/3
  From40/1 -> C18/2
  From4/1 -> Unit Delay Enabled Synchronous1/2
  From39/1 -> C17/3
  From38/1 -> C17/2
  From37/1 -> C23/3
  From36/1 -> C23/2
  From35/1 -> C22/3
  From34/1 -> C22/2
  From33/1 -> C21/3
  From32/1 -> C21/2
  From31/1 -> C13/3
  From30/1 -> C13/2
  From3/1 -> Switch1/2
  From29/1 -> C12/3
  From28/1 -> C12/2
  From27/1 -> C11/3
  From26/1 -> C11/2
  From25/1 -> C10/3
  From24/1 -> C10/2
  From23/1 -> C16/3
  From22/1 -> C16/2
  From21/1 -> C15/3
  From20/1 -> C15/2
  From2/1 -> Unit Delay Enabled Synchronous/2
  From19/1 -> C14/3
  From18/1 -> C14/2
  From17/1 -> C9/3
  From16/1 -> C9/2
  From15/1 -> C8/3
  From14/1 -> C8/2
  From13/1 -> C7/3
  From12/1 -> C7/2
  From11/1 -> C6/3
  From10/1 -> C6/2
  From1/1 -> Switch/2
  From/1 -> Unit Delay Enabled Synchronous3/2
  Delay5/1 -> Sample Control Bus Creator/3
  Delay4/1 -> Sample Control Bus Creator/2
  Delay3/1 -> Sample Control Bus Creator/1
  Delay1/1 -> Logical Operator/1
  bus_selector/3 -> Delay5/1, Goto2/1  "<valid>"
  bus_selector/2 -> Delay4/1  "<end>"
  bus_selector/1 -> Delay3/1, Goto3/1  "<start>"
  SI/1 -> t/1
  ctrl_in/1 -> bus_selector/1
  data_in/1 -> Delay1/1

== system gm_HDLPayloadFull_vs/payload_full/payload_rep ==
  data_in : Inport  OutDataTypeStr=boolean  SampleTime=0.125
  ctrl_in : Inport  Port=2  SampleTime=0.125
  data_out : Outport  SampleTime=0.125
  ctrl_out : Outport  Port=2  SampleTime=0.125
  wires:
  ctrl_in/1 -> ctrl_out/1
  data_in/1 -> data_out/1

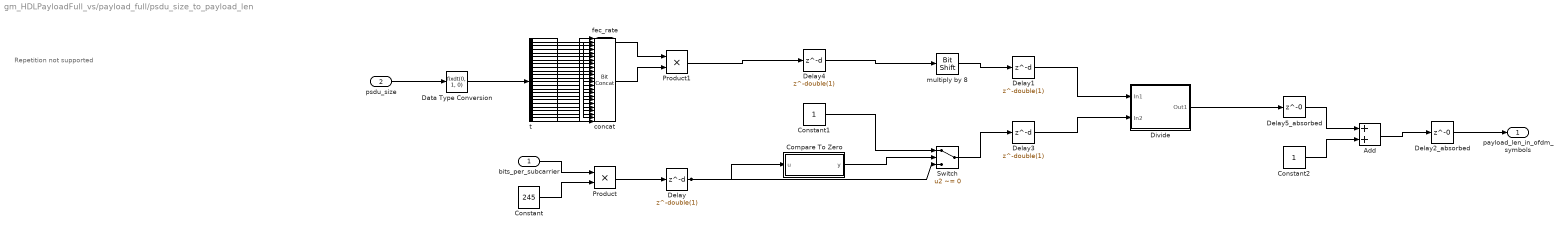
== system gm_HDLPayloadFull_vs/payload_full/psdu_size_to_payload_len ==
  note: Repetition not supported
  bits_per_subcarrier : Inport  OutDataTypeStr=fixdt(0, 4, 0)  PortDimensions=1  SampleTime=1
  psdu_size : Inport  Port=2  OutDataTypeStr=boolean  PortDimensions=[1 24]  SampleTime=1
  fec_rate : Inport  Port=3  OutDataTypeStr=fixdt(0, 4, 0)  PortDimensions=1  SampleTime=1
  Add : Sum  OutDataTypeStr=fixdt(0, 29, 0)  AccumDataTypeStr=fixdt(0, 29, 0)  SampleTime=1
  Compare To Zero : Subsystem  mask(Compare To Zero){relop===, OutDataTypeStr=boolean, ZeroCross=on}
      mask prompts: relop "Simulink:masks:Operator_MP"; OutDataTypeStr "Simulink:masks:OutputDataType_MP"; ZeroCross "Simulink:masks:EnableZerocrossingDetection_MP"
      mask help: Simulink:masks:CompareToZero_MD
      mask init:
      | OutDataTypeStr = 'boolean';
      | ZeroCross = 'on';
      | blkName = 'HDLPayloadFull/payload_full/psdu_size_to_payload_len/Compare\nTo Zero';
      | relop = '==';
      | setValue = 'boolean';
      mask TypeOptions relop: == | ~= | < | <= | >= | >
      mask TypeOptions OutDataTypeStr: Simulink:masks:uint8 | Simulink:masks:boolean
      mask Callback ZeroCross: sl('zeroCrossEnable', gcbh);
      mask Display: disp([relop,' 0'])
  Constant : Constant  Value=245  OutDataTypeStr=uint8  SampleTime=1
  Constant1 : Constant  OutDataTypeStr=fixdt(0, 12, 0)  SampleTime=1
  Constant2 : Constant  OutDataTypeStr=fixdt(0, 28, 0)  SampleTime=1
  Data Type Conversion : DataTypeConversion  OutDataTypeStr=fixdt(0, 1, 0)  SampleTime=1  SaturateOnIntegerOverflow=off  RndMeth=Floor
  Delay : Delay  DelayLength=double(1)  InitialCondition=0  SampleTime=1
  Delay1 : Delay  DelayLength=double(1)  InitialCondition=0  SampleTime=1
  Delay2_absorbed : Delay  DelayLength=0
  Delay3 : Delay  DelayLength=double(1)  InitialCondition=1  SampleTime=1
  Delay4 : Delay  DelayLength=double(1)  InitialCondition=0  SampleTime=1
  Delay5_absorbed : Delay  DelayLength=0
  Divide : Subsystem
  Product : Product  Inputs=**  OutDataTypeStr=fixdt(0, 12, 0)  SampleTime=1
  Product1 : Product  Inputs=**  OutDataTypeStr=fixdt(0, 28, 0)  SampleTime=1
  Switch : Switch  Criteria=u2 ~= 0  Threshold=double(0)  OutDataTypeStr=fixdt(0, 12, 0)  SampleTime=1  SaturateOnIntegerOverflow=off  InputSameDT=off
  concat : hdlsllib/Logic and Bit Operations/Bit Concat  numInputs=24
  multiply by 8 : hdlsllib/Logic and Bit Operations/Bit Shift  mode=Shift Left Logical  N=double(3)
  t : Demux  Outputs=24
  payload_len_in_ofdm_symbols : Outport  SampleTime=1
  wires:
  Divide/1(Out1) -> Delay5_absorbed/1
  Add/1 -> Delay2_absorbed/1
  t/24 -> concat/1
  t/23 -> concat/2
  t/22 -> concat/3
  t/21 -> concat/4
  t/20 -> concat/5
  t/19 -> concat/6
  t/18 -> concat/7
  t/17 -> concat/8
  t/16 -> concat/9
  t/15 -> concat/10
  t/14 -> concat/11
  t/13 -> concat/12
  t/12 -> concat/13
  t/11 -> concat/14
  t/10 -> concat/15
  t/9 -> concat/16
  t/8 -> concat/17
  t/7 -> concat/18
  t/6 -> concat/19
  t/5 -> concat/20
  t/4 -> concat/21
  t/3 -> concat/22
  t/2 -> concat/23
  t/1 -> concat/24
  multiply by 8/1 -> Delay1/1
  Switch/1 -> Delay3/1
  Product1/1 -> Delay4/1
  Product/1 -> Delay/1
  Delay5_absorbed/1 -> Add/1
  Delay4/1 -> multiply by 8/1
  Delay3/1 -> Divide/2(In2)
  Delay2_absorbed/1 -> payload_len_in_ofdm_symbols/1
  Delay1/1 -> Divide/1(In1)
  Delay/1 -> Compare To Zero/1(u), Switch/3
  Data Type Conversion/1 -> t/1
  Constant2/1 -> Add/2
  Constant1/1 -> Switch/1
  Constant/1 -> Product/2
  Compare To Zero/1(y) -> Switch/2
  concat/1 -> Product1/2
  fec_rate/1 -> Product1/1
  psdu_size/1 -> Data Type Conversion/1
  bits_per_subcarrier/1 -> Product/1

== system gm_HDLPayloadFull_vs/payload_full/puncturer ==
  data_in : Inport  OutDataTypeStr=boolean  SampleTime=0.125
  ctrl_in : Inport  Port=2  SampleTime=0.125
  data_out : Outport  SampleTime=0.125
  ctrl_out : Outport  Port=2  SampleTime=0.125
  wires:
  ctrl_in/1 -> ctrl_out/1
  data_in/1 -> data_out/1

== system gm_HDLPayloadFull_vs/payload_full/reduced_ldpc ==
  data_in : Inport  OutDataTypeStr=boolean  SampleTime=0.125
  ctrl_in : Inport  Port=2  SampleTime=0.125
  Hc_12S-B80 : whdledac/LDPC Encoder  ParityCheckMatrix=Hc_12S  BlockSize=80  SimulateUsing=Code generation
  data_out : Outport  SampleTime=0.125
  ctrl_out : Outport  Port=2  SampleTime=0.125
  next_frame : Outport  Port=3  SampleTime=0.125
  wires:
  Hc_12S-B80/3 -> next_frame/1
  Hc_12S-B80/2 -> ctrl_out/1
  Hc_12S-B80/1 -> data_out/1
  ctrl_in/1 -> Hc_12S-B80/2
  data_in/1 -> Hc_12S-B80/1

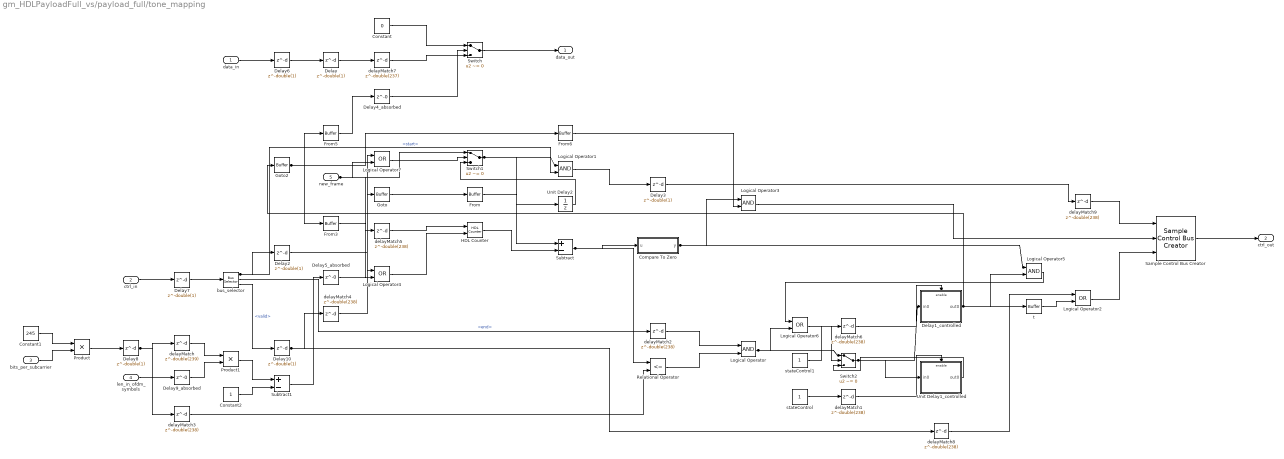
== system gm_HDLPayloadFull_vs/payload_full/tone_mapping ==
  data_in : Inport  OutDataTypeStr=boolean  SampleTime=0.125
  ctrl_in : Inport  Port=2  SampleTime=0.125
  bits_per_subcarrier : Inport  Port=3  OutDataTypeStr=fixdt(0, 4, 0)  SampleTime=0.125
  len_in_ofdm_symbols : Inport  Port=4  OutDataTypeStr=fixdt(0, 29, 0)  SampleTime=0.125
  new_frame : Inport  Port=5  OutDataTypeStr=boolean  SampleTime=0.125
  Compare To Zero : Subsystem  mask(Compare To Zero){relop===, OutDataTypeStr=boolean, ZeroCross=on}
      mask prompts: relop "Simulink:masks:Operator_MP"; OutDataTypeStr "Simulink:masks:OutputDataType_MP"; ZeroCross "Simulink:masks:EnableZerocrossingDetection_MP"
      mask help: Simulink:masks:CompareToZero_MD
      mask init:
      | OutDataTypeStr = 'boolean';
      | ZeroCross = 'on';
      | blkName = 'HDLPayloadFull/payload_full/tone_mapping/Compare\nTo Zero';
      | relop = '==';
      | setValue = 'boolean';
      mask TypeOptions relop: == | ~= | < | <= | >= | >
      mask TypeOptions OutDataTypeStr: Simulink:masks:uint8 | Simulink:masks:boolean
      mask Callback ZeroCross: sl('zeroCrossEnable', gcbh);
      mask Display: disp([relop,' 0'])
  Constant : Constant  Value=0  OutDataTypeStr=boolean  SampleTime=0.125
  Constant1 : Constant  Value=245  OutDataTypeStr=uint8  SampleTime=0.125
  Constant2 : Constant  OutDataTypeStr=fixdt(0, 41, 0)  SampleTime=0.125
  Delay{,2..3,6,8,10} (6 alike) : Delay  DelayLength=double(1)  InitialCondition=0  SampleTime=0.125
  Delay1_controlled : Subsystem
  Delay4_absorbed : Delay  DelayLength=0
  Delay5_absorbed : Delay  DelayLength=0
  Delay7 : Delay  DelayLength=double(1)  SampleTime=0.125
  Delay9_absorbed : Delay  DelayLength=0
  From{,3,5..6} (4 alike) : hdlmdlgenlib/Buffer
  Goto : hdlmdlgenlib/Buffer
  Goto2 : hdlmdlgenlib/Buffer
  HDL Counter : hdlsllib/Sources/HDL Counter  CountType=Free running  CountInit=0  CountStep=1  CountMax=numDataCarriers-1  CountFromType=Initial value  CountFrom=0  CountResetPort=on  CountLoadPort=off  CountEnbPort=on  CountDirPort=off  CountHitOutputPort=off  CountDataType=Unsigned  CountWordLen=16  CountFracLen=0  CountSampTime=1
  Logical Operator{,1,3,5} (4 alike) : Logic  AllPortsSameDT=off  OutDataTypeStr=boolean  SampleTime=0.125
  Logical Operator{2,4,6..7} (4 alike) : Logic  Operator=OR  AllPortsSameDT=off  OutDataTypeStr=boolean  SampleTime=0.125
  Product : Product  Inputs=**  OutDataTypeStr=fixdt(0, 12, 0)  SampleTime=0.125
  Product1 : Product  Inputs=**  OutDataTypeStr=fixdt(0, 41, 0)  SampleTime=0.125
  Relational Operator : RelationalOperator  Operator=<=  OutDataTypeStr=boolean  SampleTime=0.125  InputSameDT=off
  Sample Control Bus Creator : whdlutilities/Sample Control Bus Creator
  Subtract : Sum  Inputs=+-  OutDataTypeStr=fixdt(1, 43, 0)  AccumDataTypeStr=fixdt(1, 43, 0)  SampleTime=0.125
  Subtract1 : Sum  Inputs=+-  OutDataTypeStr=fixdt(1, 42, 0)  AccumDataTypeStr=fixdt(1, 42, 0)  SampleTime=0.125
  Switch : Switch  Criteria=u2 ~= 0  Threshold=double(0)  OutDataTypeStr=boolean  SampleTime=0.125  SaturateOnIntegerOverflow=off  InputSameDT=off
  Switch1 : Switch  Criteria=u2 ~= 0  Threshold=double(0)  OutDataTypeStr=boolean  SampleTime=0.125  SaturateOnIntegerOverflow=off  InputSameDT=off
  Switch2 : Switch  Criteria=u2 ~= 0  Threshold=double(0)  OutDataTypeStr=boolean  SampleTime=0.125  SaturateOnIntegerOverflow=off  InputSameDT=off
  Unit Delay1_controlled : Subsystem
  Unit Delay2 : UnitDelay  SampleTime=0.125
  bus_selector : BusSelector  OutputSignals=start,end,valid
  delayMatch : Delay  DelayLength=double(239)  InitialCondition=0  SampleTime=0.125
  delayMatch{1..6,8..9} (8 alike) : Delay  DelayLength=double(238)  InitialCondition=0  SampleTime=0.125
  delayMatch7 : Delay  DelayLength=double(237)  InitialCondition=0  SampleTime=0.125
  stateControl : Constant  OutDataTypeStr=boolean  SampleTime=0.125
  stateControl1 : Constant  OutDataTypeStr=boolean  SampleTime=0.125
  t : hdlmdlgenlib/Buffer
  data_out : Outport  SampleTime=0.125
  ctrl_out : Outport  Port=2  SampleTime=0.125
  wires:
  len_in_ofdm_symbols/1 -> Delay9_absorbed/1
  Subtract1/1 -> Delay5_absorbed/1
  Logical Operator7/1 -> Switch1/2
  Unit Delay2/1 -> Switch1/3
  Subtract/1 -> Compare To Zero/1(u), Relational Operator/1
  HDL Counter/1 -> Subtract/2
  Logical Operator4/1 -> HDL Counter/2
  From3/1 -> Logical Operator4/2
  Logical Operator/1 -> Logical Operator6/2, Switch2/1
  Relational Operator/1 -> Logical Operator/2
  Logical Operator6/1 -> Switch2/2
  Logical Operator5/1 -> Logical Operator6/1
  Switch2/1 -> Unit Delay1_controlled/1(in0), Delay1_controlled/1(in0)
  delayMatch4/1 -> Logical Operator4/1
  delayMatch3/1 -> Relational Operator/2
  delayMatch1/1 -> Unit Delay1_controlled/Enable
  delayMatch6/1 -> Delay1_controlled/Enable
  Unit Delay1_controlled/1(out0) -> Switch2/3
  Compare To Zero/1(y) -> Logical Operator3/1, Logical Operator5/1
  Delay1_controlled/1(out0) -> Logical Operator5/2, Goto2/1, t/1
  Goto2/1 -> From5/1, From6/1, From3/1
  Delay3/1 -> delayMatch9/1
  Delay10/1 -> delayMatch4/1, delayMatch8/1
  Delay/1 -> delayMatch7/1
  stateControl1/1 -> delayMatch6/1
  new_frame/1 -> Switch1/1, Logical Operator7/2, delayMatch5/1
  delayMatch8/1 -> Logical Operator2/1
  Delay8/1 -> delayMatch/1, delayMatch3/1
  bus_selector/2 -> delayMatch2/1  "<end>"
  stateControl/1 -> delayMatch1/1
  Goto/1 -> From/1
  Switch1/1 -> Unit Delay2/1, Logical Operator1/1
  Switch/1 -> data_out/1
  bus_selector/3 -> Delay10/1  "<valid>"
  delayMatch2/1 -> Logical Operator/1
  bus_selector/1 -> Delay2/1, Logical Operator1/2  "<start>"
  Sample Control Bus Creator/1 -> ctrl_out/1
  Product1/1 -> Subtract1/1
  Product/1 -> Delay8/1
  Logical Operator3/1 -> Sample Control Bus Creator/2
  Logical Operator2/1 -> Sample Control Bus Creator/3
  Logical Operator1/1 -> Delay3/1
  From6/1 -> Logical Operator3/2
  From5/1 -> Delay4_absorbed/1
  From/1 -> Subtract/1
  Delay9_absorbed/1 -> Product1/2
  delayMatch/1 -> Product1/1
  Delay7/1 -> bus_selector/1
  Delay6/1 -> Delay/1
  Delay5_absorbed/1 -> Goto/1
  Delay4_absorbed/1 -> Switch/2
  delayMatch9/1 -> Sample Control Bus Creator/1
  Delay2/1 -> Logical Operator7/1
  t/1 -> Logical Operator2/2
  delayMatch7/1 -> Switch/3
  Constant2/1 -> Subtract1/2
  Constant1/1 -> Product/1
  Constant/1 -> Switch/1
  delayMatch5/1 -> HDL Counter/1
  bits_per_subcarrier/1 -> Product/2
  ctrl_in/1 -> Delay7/1
  data_in/1 -> Delay6/1

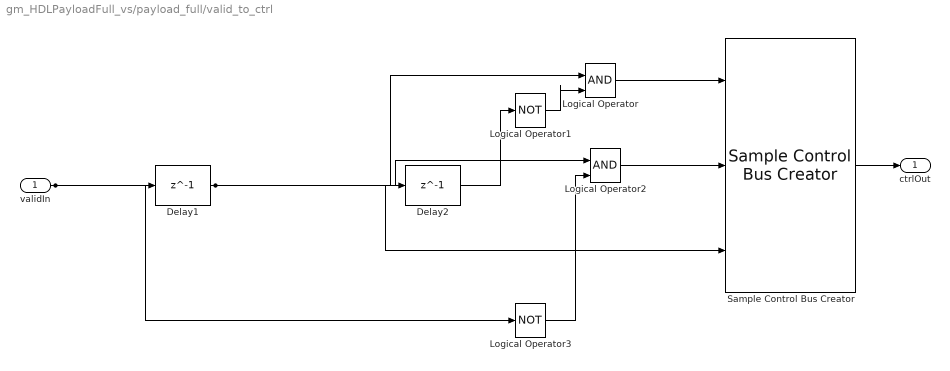
== system gm_HDLPayloadFull_vs/payload_full/valid_to_ctrl ==
  validIn : Inport  OutDataTypeStr=boolean  SampleTime=0.125
  Delay1 : Delay  DelayLength=1  InitialCondition=0  UseCircularBuffer=on
  Delay2 : Delay  DelayLength=1  InitialCondition=0  UseCircularBuffer=on
  Logical Operator : Logic  IconShape=distinctive  AllPortsSameDT=off  OutDataTypeStr=boolean
  Logical Operator1 : Logic  Operator=NOT  IconShape=distinctive  AllPortsSameDT=off  OutDataTypeStr=boolean
  Logical Operator2 : Logic  IconShape=distinctive  AllPortsSameDT=off  OutDataTypeStr=boolean
  Logical Operator3 : Logic  Operator=NOT  IconShape=distinctive  AllPortsSameDT=off  OutDataTypeStr=boolean
  Sample Control Bus Creator : whdlutilities/Sample Control Bus Creator
  ctrlOut : Outport  SampleTime=0.125
  wires:
  Sample Control Bus Creator/1 -> ctrlOut/1
  Logical Operator3/1 -> Logical Operator2/2
  Logical Operator2/1 -> Sample Control Bus Creator/2
  Logical Operator1/1 -> Logical Operator/2
  Logical Operator/1 -> Sample Control Bus Creator/1
  Delay2/1 -> Logical Operator1/1
  Delay1/1 -> Sample Control Bus Creator/3, Delay2/1, Logical Operator/1, Logical Operator2/1
  validIn/1 -> Delay1/1, Logical Operator3/1

== system gm_HDLPayloadFull_vs/payload_full/next_frame_to_ready/rising_edge_detector ==
  In : Inport  OutDataTypeStr=boolean  SampleTime=1
  Delay2 : Delay  DelayLength=1  InitialCondition=0  UseCircularBuffer=on
  Logical Operator1 : Logic  IconShape=distinctive  AllPortsSameDT=off  OutDataTypeStr=boolean
  Logical Operator2 : Logic  Operator=NOT  IconShape=distinctive  AllPortsSameDT=off  OutDataTypeStr=boolean
  Out : Outport  SampleTime=1
  wires:
  Logical Operator2/1 -> Logical Operator1/2
  Logical Operator1/1 -> Out/1
  Delay2/1 -> Logical Operator2/1
  In/1 -> Delay2/1, Logical Operator1/1

== system gm_HDLPayloadFull_vs/payload_full/psdu_size_to_payload_len/Compare To Zero ==
  u : Inport  OutDataTypeStr=fixdt(0, 12, 0)  SampleTime=1
  Compare : RelationalOperator  Operator===  OutDataTypeStr=boolean
  Constant : Constant  DisableCoverage=on  Value=0  OutDataTypeStr=fixdt(0, 12, 0)  SampleTime=-1  PreserveConstantTs=on
  y : Outport  SampleTime=1
  wires:
  Constant/1 -> Compare/2
  Compare/1 -> y/1
  u/1 -> Compare/1

== system gm_HDLPayloadFull_vs/payload_full/psdu_size_to_payload_len/Divide ==
  In1 : Inport
  In2 : Inport  Port=2
  Divide : Product  Inputs=*/  OutDataTypeStr=fixdt(0, 28, 0)  RndMeth=Zero  SaturateOnIntegerOverflow=on
  Divide_pd1 : Delay  DelayLength=32
  Out1 : Outport
  wires:
  In1/1 -> Divide/1
  In2/1 -> Divide/2
  Divide/1 -> Divide_pd1/1
  Divide_pd1/1 -> Out1/1

== system gm_HDLPayloadFull_vs/payload_full/tone_mapping/Compare To Zero ==
  u : Inport  OutDataTypeStr=fixdt(1, 43, 0)  SampleTime=0.125
  Compare : RelationalOperator  Operator===  OutDataTypeStr=boolean
  Constant : Constant  DisableCoverage=on  Value=0  OutDataTypeStr=fixdt(1, 43, 0)  SampleTime=-1  PreserveConstantTs=on
  y : Outport  SampleTime=0.125
  wires:
  Constant/1 -> Compare/2
  Compare/1 -> y/1
  u/1 -> Compare/1

== system gm_HDLPayloadFull_vs/payload_full/tone_mapping/Delay1_controlled ==
  in0 : Inport  OutDataTypeStr=boolean  SampleTime=0.125
  stateControl : EnablePort  OutDataTypeStr=boolean
  Delay1 : Delay  DelayLength=double(1)  InitialCondition=0  SampleTime=0.125
  out0 : Outport  OutDataTypeStr=boolean  SampleTime=0.125
  wires:
  in0/1 -> Delay1/1
  Delay1/1 -> out0/1

== system gm_HDLPayloadFull_vs/payload_full/tone_mapping/Unit Delay1_controlled ==
  in0 : Inport  OutDataTypeStr=boolean  SampleTime=0.125
  stateControl : EnablePort  OutDataTypeStr=boolean
  Unit Delay1 : UnitDelay  SampleTime=0.125
  out0 : Outport  OutDataTypeStr=boolean  SampleTime=0.125
  wires:
  in0/1 -> Unit Delay1/1
  Unit Delay1/1 -> out0/1
